simulink model "Hall_Sensors"  (R2023a)
settings: Solver=VariableStepAuto  StartTime=0.0  StopTime=10.0  RelTol=1e-3
settings Model: Creator=Artem Sannikov  LastModifiedBy=Artem Sannikov

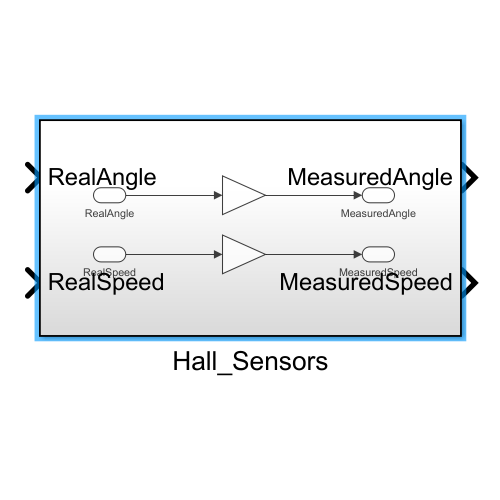
[thumbnail: Simulink's stored preview of the top-level diagram]
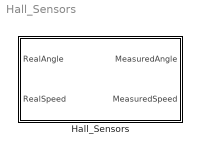
== system Hall_Sensors ==
  Hall_Sensors : Subsystem

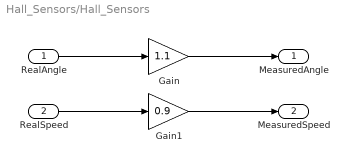
== system Hall_Sensors/Hall_Sensors ==
  RealAngle : Inport
  RealSpeed : Inport  Port=2
  Gain : Gain  Gain=1.1
  Gain1 : Gain  Gain=0.9
  MeasuredAngle : Outport
  MeasuredSpeed : Outport  Port=2
  wires:
  RealAngle/1 -> Gain/1
  Gain/1 -> MeasuredAngle/1
  RealSpeed/1 -> Gain1/1
  Gain1/1 -> MeasuredSpeed/1
